simulink model "Exercise2SIM"  (R2025b)
settings: Solver=VariableStepAuto  StartTime=0.0  StopTime=80  RelTol=1e-3
values from neighbouring files (symbols this model uses):
  A = [   0,                                        1,            0,                                              0,    0 ... (first row only)    [Exercise1.m]    (also in Exercise_2.m = [   0,  1,           0,  0,    0; symbolic_state_space_gen.m = jacobian(dx, x))
  B = [                           0 ... (first row only)    [Exercise1.m]    (also in Exercise_2.m = [0,     0; symbolic_state_space_gen.m = jacobian(dx, u))
  C = [-K/ms, -(2*zeta0*(K*ms)^(1/2) + 2*zeta_d*(K*ms)^(1/2))/ms, K/ms, (2*zeta0*(K*ms)^(1/2) - 2*zeta_d*(K*ms)^(1/2))/ms, 0 ... (first row only)    [Exercise1.m]    (also in Exercise_2.m = [-K/ms, 0, K/ms, 0, 0; symbolic_state_space_gen.m = jacobian(y, x))
  D = [                        0 ... (first row only)    [Exercise1.m]    (also in Exercise_2.m = [0, 1/ms; symbolic_state_space_gen.m = jacobian(y, u))
  V = 20    [Exercise_2.m]
libraries: simulink x1
settings Model: Creator=Alberto  LastModifiedBy=denni
settings OptimizationCC: ReuseModelBlockBuffer=off
settings RTWCC: GPUComputeCapability=3.5

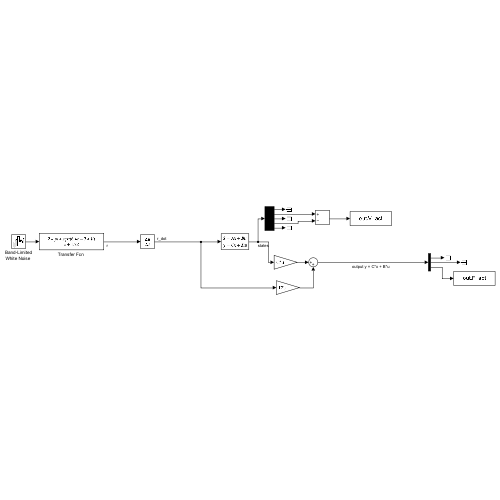
[thumbnail: Simulink's stored preview of the top-level diagram]
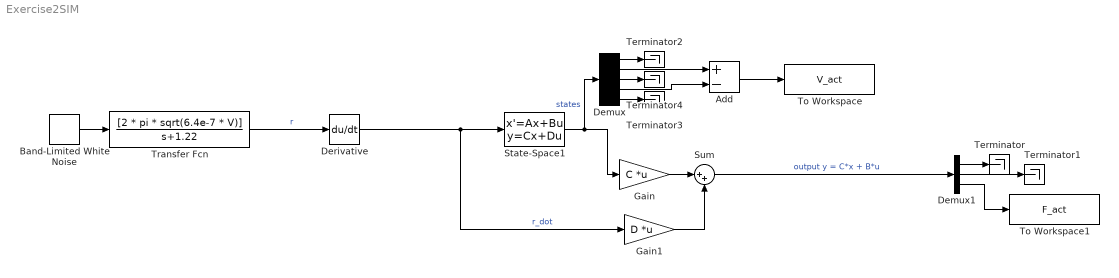
== system Exercise2SIM ==
  Add : Sum  Inputs=+-
  "Band-Limited White Noise " : simulink/Sources/Band-Limited White Noise  Cov=1  Ts=0.05  seed=0019234
  Demux : Demux  Outputs=5
  Demux1 : Demux  Outputs=3
  Derivative : Derivative
  Gain : Gain  Gain=C  Multiplication=Matrix(K*u)
  Gain1 : Gain  Gain=D  Multiplication=Matrix(K*u)
  State-Space1 : StateSpace  A=A  B=B  C=eye(5)  D=zeros(5,1)  InitialCondition=0
  Sum : Sum  Inputs=|++
  Terminator{,1..4} (5 alike) : Terminator
  To Workspace : ToWorkspace  VariableName=V_act  SampleTime=-1
  To Workspace1 : ToWorkspace  VariableName=F_act  SampleTime=-1
  "Transfer Fcn " : TransferFcn  Numerator=[2 * pi * sqrt(6.4e-7 * V)]  Denominator=[1 1.22]
  wires:
  "Band-Limited White Noise "/1 -> "Transfer Fcn "/1
  Derivative/1 -> Gain1/1, State-Space1/1  "r_dot"
  Sum/1 -> Demux1/1  "output y = C*x + B*u"
  State-Space1/1 -> Demux/1, Gain/1  "states"
  Gain/1 -> Sum/1
  Gain1/1 -> Sum/2
  Demux/2 -> Add/1
  Demux/4 -> Add/2
  Add/1 -> To Workspace/1
  Demux1/3 -> To Workspace1/1
  "Transfer Fcn "/1 -> Derivative/1  "r"
  Demux1/1 -> Terminator/1
  Demux1/2 -> Terminator1/1
  Demux/1 -> Terminator2/1
  Demux/5 -> Terminator3/1
  Demux/3 -> Terminator4/1
